simulink library "lib_Convection_FCHorizPlate"  (R2015a)
settings: Solver=ode45  StartTime=0.0  StopTime=10.0  RelTol=1e-3
libraries: simulink x21, lib_GenTools_MinMax x1
settings Model: Creator=jlkratz  LastModifiedBy=jlkratz

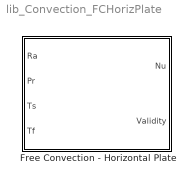
== system lib_Convection_FCHorizPlate ==
  Free Convection - Horizontal Plate : Subsystem  mask(TSAT: Horizontal Plate Free Convection){UpperOrLower_M=off}
      mask prompts: UpperOrLower_M "UpperOrLower_M - Checked for the upper surface of the plate, unchecked for the lower surface"
      mask help:
      | This block estimates the average Nusselt number of free convection on the surface of a horizontal plate.  Note that all fluid properrties should be evaluated at film temperature (average of the bulk fluid and surface temperatures). Also note that the charateristic length used to calculate the Rayleigh number should be consistent with recommendation for the shape of the plate. It has been shown that for a variety of shapes the characteristic length can be defined as L = A/P, where A is the area of the plate (one side) and P is it's perimeter. Flow patterns and heat transfer are heavily dependent on whether the plate is hot or cold and whether the surface is on the top or the bottom. This block employs different correlations to handle each case.
      |
      | For more information see the block help menu.
      mask Help: web(which('Convection_TSAT_FCHorizPlate.html'),'-helpbrowser')

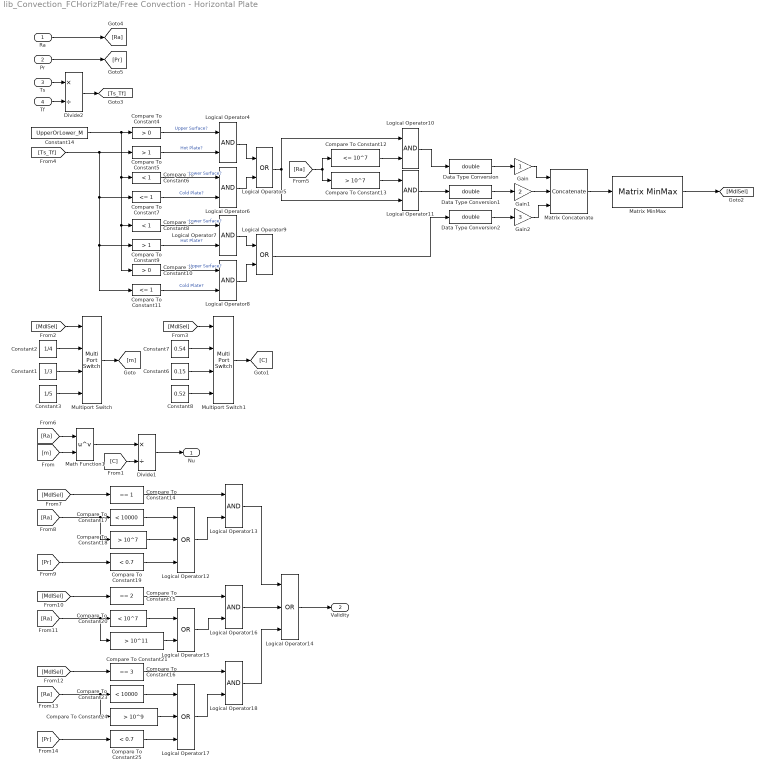
== system lib_Convection_FCHorizPlate/Free Convection - Horizontal Plate ==
  Ra : Inport
  Pr : Inport  Port=2
  Ts : Inport  Port=3
  Tf : Inport  Port=4
  Compare To Constant10 : simulink/Logic and Bit Operations/Compare To Constant  relop=>  const=0  OutDataTypeStr=boolean
  Compare To Constant11 : simulink/Logic and Bit Operations/Compare To Constant  relop=<=  const=1  OutDataTypeStr=boolean
  Compare To Constant12 : simulink/Logic and Bit Operations/Compare To Constant  relop=<=  const=10^7  OutDataTypeStr=boolean
  Compare To Constant13 : simulink/Logic and Bit Operations/Compare To Constant  relop=>  const=10^7  OutDataTypeStr=boolean
  Compare To Constant14 : simulink/Logic and Bit Operations/Compare To Constant  relop===  const=1  OutDataTypeStr=boolean
  Compare To Constant15 : simulink/Logic and Bit Operations/Compare To Constant  relop===  const=2  OutDataTypeStr=boolean
  Compare To Constant16 : simulink/Logic and Bit Operations/Compare To Constant  relop===  const=3  OutDataTypeStr=boolean
  Compare To Constant17 : simulink/Logic and Bit Operations/Compare To Constant  relop=<  const=10000  OutDataTypeStr=boolean
  Compare To Constant18 : simulink/Logic and Bit Operations/Compare To Constant  relop=>  const=10^7  OutDataTypeStr=boolean
  Compare To Constant19 : simulink/Logic and Bit Operations/Compare To Constant  relop=<  const=0.7  OutDataTypeStr=boolean
  Compare To Constant20 : simulink/Logic and Bit Operations/Compare To Constant  relop=<  const=10^7  OutDataTypeStr=boolean
  Compare To Constant21 : simulink/Logic and Bit Operations/Compare To Constant  relop=>  const=10^11  OutDataTypeStr=boolean
  Compare To Constant23 : simulink/Logic and Bit Operations/Compare To Constant  relop=<  const=10000  OutDataTypeStr=boolean
  Compare To Constant24 : simulink/Logic and Bit Operations/Compare To Constant  relop=>  const=10^9  OutDataTypeStr=boolean
  Compare To Constant25 : simulink/Logic and Bit Operations/Compare To Constant  relop=<  const=0.7  OutDataTypeStr=boolean
  Compare To Constant4 : simulink/Logic and Bit Operations/Compare To Constant  relop=>  const=0  OutDataTypeStr=boolean
  Compare To Constant5 : simulink/Logic and Bit Operations/Compare To Constant  relop=>  const=1  OutDataTypeStr=boolean
  Compare To Constant6 : simulink/Logic and Bit Operations/Compare To Constant  relop=<  const=1  OutDataTypeStr=boolean
  Compare To Constant7 : simulink/Logic and Bit Operations/Compare To Constant  relop=<=  const=1  OutDataTypeStr=boolean
  Compare To Constant8 : simulink/Logic and Bit Operations/Compare To Constant  relop=<  const=1  OutDataTypeStr=boolean
  Compare To Constant9 : simulink/Logic and Bit Operations/Compare To Constant  relop=>  const=1  OutDataTypeStr=boolean
  Constant1 : Constant  Value=1/3
  Constant14 : Constant  Value=UpperOrLower_M
  Constant2 : Constant  Value=1/4
  Constant3 : Constant  Value=1/5
  Constant6 : Constant  Value=0.15
  Constant7 : Constant  Value=0.54
  Constant8 : Constant  Value=0.52
  Data Type Conversion : DataTypeConversion  OutDataTypeStr=double
  Data Type Conversion1 : DataTypeConversion  OutDataTypeStr=double
  Data Type Conversion2 : DataTypeConversion  OutDataTypeStr=double
  Divide1 : Product  Inputs=*/
  Divide2 : Product  Inputs=*/
  Gain : Gain
  Gain1 : Gain  Gain=2
  Gain2 : Gain  Gain=3
  Logical Operator{4,6..8,10..11,13,16,18} (9 alike) : Logic  AllPortsSameDT=off  OutDataTypeStr=boolean
  Logical Operator12 : Logic  Operator=OR  Inputs=3  AllPortsSameDT=off  OutDataTypeStr=boolean
  Logical Operator14 : Logic  Operator=OR  Inputs=3  AllPortsSameDT=off  OutDataTypeStr=boolean
  Logical Operator15 : Logic  Operator=OR  AllPortsSameDT=off  OutDataTypeStr=boolean
  Logical Operator17 : Logic  Operator=OR  Inputs=3  AllPortsSameDT=off  OutDataTypeStr=boolean
  Logical Operator5 : Logic  Operator=OR  AllPortsSameDT=off  OutDataTypeStr=boolean
  Logical Operator9 : Logic  Operator=OR  AllPortsSameDT=off  OutDataTypeStr=boolean
  Math Function1 : Math  Operator=pow  SaturateOnIntegerOverflow=on
  Matrix Concatenate : Concatenate  NumInputs=3  Mode=Multidimensional array  ConcatenateDimension=2
  Matrix MinMax : lib_GenTools_MinMax/Matrix MinMax  rows_M=on  cols_M=off  all_M=off  minmax_M=off  BN_M=gcb
  Multiport Switch : MultiPortSwitch
  Multiport Switch1 : MultiPortSwitch
  Nu : Outport
  Validity : Outport  Port=2
  wires:
  Matrix Concatenate/1 -> Matrix MinMax/1
  Logical Operator18/1 -> Logical Operator14/3
  Logical Operator16/1 -> Logical Operator14/2
  Logical Operator13/1 -> Logical Operator14/1
  Logical Operator17/1 -> Logical Operator18/2
  Compare To Constant16/1 -> Logical Operator18/1
  Compare To Constant25/1 -> Logical Operator17/3
  Compare To Constant24/1 -> Logical Operator17/2
  Compare To Constant23/1 -> Logical Operator17/1
  [Pr] -> Compare To Constant25/1
  [Ra] -> Compare To Constant24/1, Compare To Constant23/1
  [MdlSel] -> Compare To Constant16/1
  Logical Operator15/1 -> Logical Operator16/2
  Compare To Constant15/1 -> Logical Operator16/1
  Compare To Constant21/1 -> Logical Operator15/2
  Compare To Constant20/1 -> Logical Operator15/1
  [Ra] -> Compare To Constant21/1, Compare To Constant20/1
  [MdlSel] -> Compare To Constant15/1
  Logical Operator12/1 -> Logical Operator13/2
  Compare To Constant14/1 -> Logical Operator13/1
  Compare To Constant19/1 -> Logical Operator12/3
  Compare To Constant18/1 -> Logical Operator12/2
  Compare To Constant17/1 -> Logical Operator12/1
  [Pr] -> Compare To Constant19/1
  [Ra] -> Compare To Constant17/1, Compare To Constant18/1
  [MdlSel] -> Compare To Constant14/1
  Divide1/1 -> Nu/1
  [C] -> Divide1/2
  [m] -> Math Function1/2
  Math Function1/1 -> Divide1/1
  [Ra] -> Math Function1/1
  Pr/1 -> [Pr]
  Logical Operator10/1 -> Data Type Conversion/1
  Logical Operator11/1 -> Data Type Conversion1/1
  Logical Operator5/1 -> Logical Operator10/1, Logical Operator11/2
  Compare To Constant12/1 -> Logical Operator10/2
  Compare To Constant13/1 -> Logical Operator11/1
  [Ra] -> Compare To Constant12/1, Compare To Constant13/1
  Logical Operator9/1 -> Data Type Conversion2/1
  Logical Operator8/1 -> Logical Operator9/2
  Logical Operator7/1 -> Logical Operator9/1
  Gain2/1 -> Matrix Concatenate/3
  Gain1/1 -> Matrix Concatenate/2
  Gain/1 -> Matrix Concatenate/1
  Compare To Constant11/1 -> Logical Operator8/2  "Cold Plate?"
  Compare To Constant10/1 -> Logical Operator8/1  "Upper Surface?"
  Compare To Constant9/1 -> Logical Operator7/2  "Hot Plate?"
  Compare To Constant8/1 -> Logical Operator7/1  "Lower Surface?"
  Logical Operator4/1 -> Logical Operator5/1
  Logical Operator6/1 -> Logical Operator5/2
  Compare To Constant7/1 -> Logical Operator6/2  "Cold Plate?"
  Compare To Constant6/1 -> Logical Operator6/1  "Lower Surface?"
  Compare To Constant5/1 -> Logical Operator4/2  "Hot Plate?"
  Compare To Constant4/1 -> Logical Operator4/1  "Upper Surface?"
  [Ts_Tf] -> Compare To Constant5/1, Compare To Constant11/1, Compare To Constant9/1, Compare To Constant7/1
  Constant14/1 -> Compare To Constant4/1, Compare To Constant6/1, Compare To Constant8/1, Compare To Constant10/1
  Data Type Conversion/1 -> Gain/1
  Data Type Conversion1/1 -> Gain1/1
  Data Type Conversion2/1 -> Gain2/1
  Matrix MinMax/1 -> [MdlSel]
  [MdlSel] -> Multiport Switch1/1
  [MdlSel] -> Multiport Switch/1
  Multiport Switch1/1 -> [C]
  Constant7/1 -> Multiport Switch1/2
  Constant6/1 -> Multiport Switch1/3
  Constant8/1 -> Multiport Switch1/4
  Multiport Switch/1 -> [m]
  Constant2/1 -> Multiport Switch/2
  Constant1/1 -> Multiport Switch/3
  Constant3/1 -> Multiport Switch/4
  Divide2/1 -> [Ts_Tf]
  Tf/1 -> Divide2/2
  Ts/1 -> Divide2/1
  Logical Operator14/1 -> Validity/1
  Ra/1 -> [Ra]
